simulink model "simulation"  (R2024b)
settings: Solver=ode4  StartTime=0.0  StopTime=10  FixedStep=0.001  RelTol=1e-3
settings Model: Creator=yagiz  LastModifiedBy=yagiz

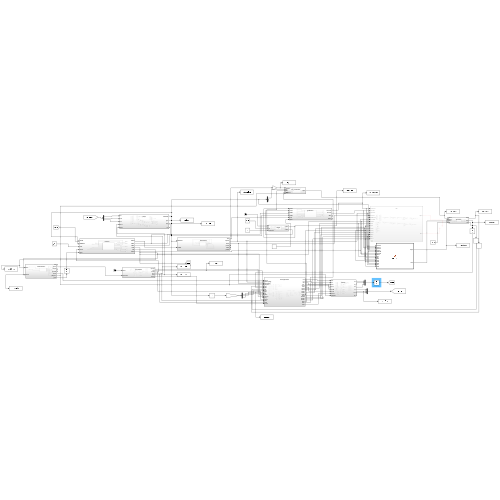
[thumbnail: Simulink's stored preview of the top-level diagram]
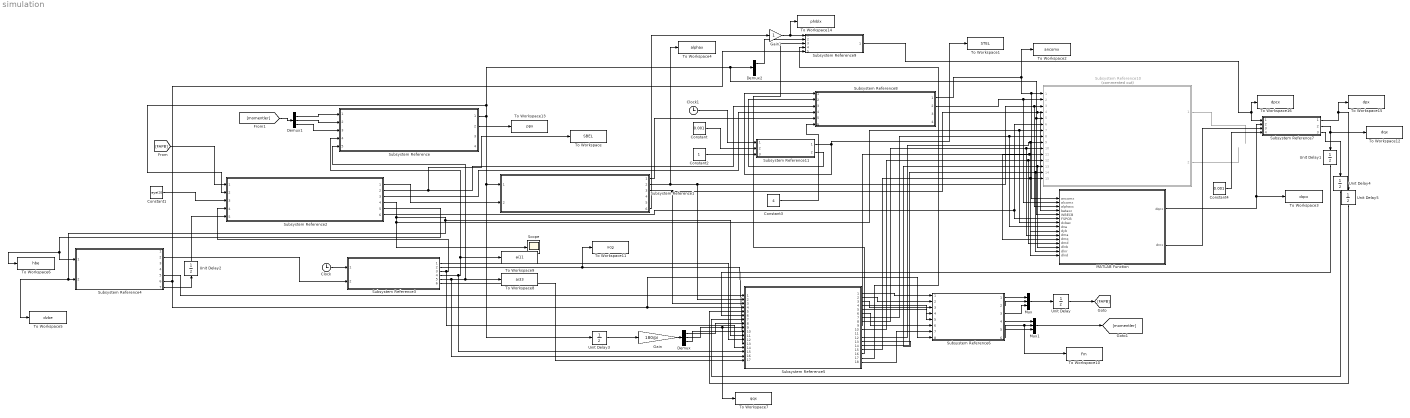
== system simulation ==
  Clock : Clock
  Clock1 : Clock
  Constant : Constant  Value=0.001
  Constant1 : Constant  Value=eye(3)
  Constant2 : Constant
  Constant3 : Constant  Value=4
  Constant4 : Constant  Value=0.001
  Demux : Demux  Outputs=3
  Demux1 : Demux  Outputs=3
  Demux2 : Demux  Outputs=3
  Gain : Gain  Gain=180/pi
  Gain1 : Gain
  MATLAB Function : MATLAB Function  TreatAsAtomicUnit=on
  Mux : Mux  Inputs=3
  Mux1 : Mux  Inputs=3
  Scope : Scope
  Subsystem Reference : Subsystem  ReferencedSubsystem=euler
  Subsystem Reference1 : Subsystem  ReferencedSubsystem=kinematics
  Subsystem Reference10 : Subsystem  Commented=on  ReferencedSubsystem=ndi
  Subsystem Reference11 : Subsystem  ReferencedSubsystem=target
  Subsystem Reference2 : Subsystem  ReferencedSubsystem=newton
  Subsystem Reference3 : Subsystem  ReferencedSubsystem=propulsion
  Subsystem Reference4 : Subsystem  ReferencedSubsystem=environment
  Subsystem Reference5 : Subsystem  ReferencedSubsystem=aerodynamics
  Subsystem Reference6 : Subsystem  ReferencedSubsystem=forces
  Subsystem Reference7 : Subsystem  ReferencedSubsystem=actuator
  Subsystem Reference8 : Subsystem  ReferencedSubsystem=guidance
  Subsystem Reference9 : Subsystem  ReferencedSubsystem=roll_controller
  To Workspace : ToWorkspace  VariableName=SBEL  SaveFormat=Timeseries  SampleTime=-1
  To Workspace1 : ToWorkspace  VariableName=STEL  SaveFormat=Timeseries  SampleTime=-1
  To Workspace10 : ToWorkspace  VariableName=Fm  SaveFormat=Timeseries  SampleTime=-1
  To Workspace11 : ToWorkspace  VariableName=xcg  SaveFormat=Timeseries  SampleTime=-1
  To Workspace12 : ToWorkspace  VariableName=dqx  SaveFormat=Timeseries  SampleTime=-1
  To Workspace13 : ToWorkspace  VariableName=ppx  SaveFormat=Timeseries  SampleTime=-1
  To Workspace14 : ToWorkspace  VariableName=phiblx  SaveFormat=Timeseries  SampleTime=-1
  To Workspace15 : ToWorkspace  VariableName=dpx  SaveFormat=Timeseries  SampleTime=-1
  To Workspace16 : ToWorkspace  VariableName=dpcx  SaveFormat=Timeseries  SampleTime=-1
  To Workspace2 : ToWorkspace  VariableName=ancomx  SaveFormat=Timeseries  SampleTime=-1
  To Workspace3 : ToWorkspace  VariableName=dqcx  SaveFormat=Timeseries  SampleTime=-1
  To Workspace4 : ToWorkspace  VariableName=alphax  SaveFormat=Timeseries  SampleTime=-1
  To Workspace5 : ToWorkspace  VariableName=dvbe  SaveFormat=Timeseries  SampleTime=-1
  To Workspace6 : ToWorkspace  VariableName=hbe  SaveFormat=Timeseries  SampleTime=-1
  To Workspace7 : ToWorkspace  VariableName=qqx  SaveFormat=Timeseries  SampleTime=-1
  To Workspace8 : ToWorkspace  VariableName=ai33  SaveFormat=Timeseries  SampleTime=-1
  To Workspace9 : ToWorkspace  VariableName=ai11  SaveFormat=Timeseries  SampleTime=-1
  Unit Delay : UnitDelay  InitialCondition=[0;0;0]  SampleTime=0.001  HasFrameUpgradeWarning=on
  Unit Delay1 : UnitDelay  SampleTime=0.001  HasFrameUpgradeWarning=on
  Unit Delay2 : UnitDelay  InitialCondition=9.8065  SampleTime=0.001  HasFrameUpgradeWarning=on
  Unit Delay3 : UnitDelay  InitialCondition=[0;0;0]  SampleTime=0.001  HasFrameUpgradeWarning=on
  Unit Delay4 : UnitDelay  SampleTime=0.001  HasFrameUpgradeWarning=on
  Unit Delay5 : UnitDelay  SampleTime=0.001  HasFrameUpgradeWarning=on
  wires:
  Constant1/1 -> Subsystem Reference2/3
  Subsystem Reference2/1 -> Subsystem Reference1/2
  Clock/1 -> Subsystem Reference3/1
  Subsystem Reference3/3 -> Subsystem Reference5/14, Subsystem Reference2/4
  Subsystem Reference3/4 -> Subsystem Reference5/15, Subsystem Reference/4, To Workspace9/1
  Subsystem Reference3/5 -> Subsystem Reference5/16, Subsystem Reference/5, To Workspace8/1
  Subsystem Reference4/2 -> Subsystem Reference3/2
  Subsystem Reference4/7 -> Unit Delay2/1
  Subsystem Reference4/5 -> Subsystem Reference5/1
  Subsystem Reference4/6 -> Subsystem Reference9/5, Subsystem Reference6/8, Subsystem Reference5/4
  Subsystem Reference1/2 -> Subsystem Reference5/2, MATLAB Function/3(alphaxc), Subsystem Reference10/3, To Workspace4/1
  Subsystem Reference1/3 -> Subsystem Reference5/3, MATLAB Function/4(betaxc), Subsystem Reference10/4
  Subsystem Reference3/6 -> Subsystem Reference5/17
  Gain/1 -> Demux/1
  Demux/1 -> Subsystem Reference5/8
  Demux/2 -> To Workspace7/1, Subsystem Reference5/9
  Demux/3 -> Subsystem Reference5/10
  Subsystem Reference3/1 -> Subsystem Reference5/12
  Subsystem Reference3/2 -> Subsystem Reference5/13, To Workspace11/1
  Subsystem Reference5/1 -> Subsystem Reference6/1
  Subsystem Reference5/2 -> Subsystem Reference6/2
  Subsystem Reference5/3 -> Subsystem Reference6/3
  Subsystem Reference5/4 -> Subsystem Reference6/4
  Subsystem Reference5/5 -> Subsystem Reference6/5
  Subsystem Reference5/6 -> Subsystem Reference6/6
  Subsystem Reference5/18 -> Subsystem Reference6/7
  Subsystem Reference6/1 -> Mux/1
  Subsystem Reference6/2 -> Mux/2
  Subsystem Reference6/3 -> Mux/3
  Mux/1 -> Unit Delay/1
  Subsystem Reference6/4 -> Mux1/1
  Subsystem Reference6/5 -> To Workspace10/1, Mux1/2
  Subsystem Reference6/6 -> Mux1/3
  [FAPB] -> Subsystem Reference2/1
  [momentler] -> Demux1/1
  Demux1/1 -> Subsystem Reference/1
  Demux1/2 -> Subsystem Reference/2
  Demux1/3 -> Subsystem Reference/3
  Subsystem Reference2/5 -> To Workspace6/1, Subsystem Reference4/1
  Unit Delay/1 -> [FAPB]
  Mux1/1 -> [momentler]
  Unit Delay2/1 -> Subsystem Reference2/5
  Subsystem Reference2/4 -> Scope/1, Subsystem Reference10/7, MATLAB Function/7(dvbec), Subsystem Reference5/11, To Workspace5/1, Subsystem Reference4/2
  Clock1/1 -> Subsystem Reference11/1
  Constant/1 -> Subsystem Reference11/2
  Constant2/1 -> Subsystem Reference11/3
  Subsystem Reference11/1 -> To Workspace1/1, Subsystem Reference8/1
  Subsystem Reference11/2 -> Subsystem Reference8/2
  Constant3/1 -> Subsystem Reference8/6
  Subsystem Reference1/1 -> Subsystem Reference8/5
  Subsystem Reference2/2 -> To Workspace/1, Subsystem Reference8/3
  Subsystem Reference2/3 -> Subsystem Reference8/4
  Subsystem Reference1/6 -> Gain1/1
  Subsystem Reference10/1 -> ?
  Subsystem Reference10/2 -> ?
  Subsystem Reference7/1 -> Unit Delay5/1, To Workspace15/1
  Subsystem Reference7/2 -> To Workspace12/1, Unit Delay1/1
  Subsystem Reference7/3 -> Unit Delay4/1
  Constant4/1 -> Subsystem Reference7/4
  Subsystem Reference8/1 -> To Workspace2/1, MATLAB Function/1(ancomx), Subsystem Reference10/1
  Subsystem Reference8/2 -> MATLAB Function/2(alcomx), Subsystem Reference10/2
  Subsystem Reference5/16 -> Subsystem Reference9/3
  Subsystem Reference5/17 -> Subsystem Reference9/4
  Subsystem Reference5/7 -> Subsystem Reference10/8, MATLAB Function/8(dna)
  Subsystem Reference5/12 -> MATLAB Function/9(dyb), Subsystem Reference10/9
  Subsystem Reference5/8 -> MATLAB Function/10(dma), Subsystem Reference10/10
  Subsystem Reference5/9 -> MATLAB Function/11(dmq), Subsystem Reference10/11
  Subsystem Reference5/10 -> MATLAB Function/12(dmd), Subsystem Reference10/12
  Subsystem Reference5/13 -> MATLAB Function/13(dlnb), Subsystem Reference10/13
  Subsystem Reference5/14 -> MATLAB Function/14(dlnr), Subsystem Reference10/14
  Subsystem Reference5/15 -> MATLAB Function/15(dlnd), Subsystem Reference10/15
  Subsystem Reference/1 -> MATLAB Function/5(WBECB), Subsystem Reference10/5, Demux2/1, Subsystem Reference2/2, Unit Delay3/1, Subsystem Reference1/1
  Subsystem Reference2/6 -> Subsystem Reference10/6, MATLAB Function/6(FSPCB)
  MATLAB Function/1(dqcx) -> Subsystem Reference7/2, To Workspace3/1
  MATLAB Function/2(drcx) -> Subsystem Reference7/3
  Unit Delay3/1 -> Gain/1
  Subsystem Reference/2 -> To Workspace13/1
  Subsystem Reference9/1 -> To Workspace16/1, Subsystem Reference7/1
  Demux2/1 -> Subsystem Reference9/2
  Gain1/1 -> To Workspace14/1, Subsystem Reference9/1
  Unit Delay1/1 -> Subsystem Reference5/6
  Unit Delay4/1 -> Subsystem Reference5/7
  Unit Delay5/1 -> Subsystem Reference5/5

== matlab function simulation/MATLAB Function ==
  data: ancomx input; dqcx output; alcomx input; alphaxc input; betaxc input; WBECB input; FSPCB input; dvbec input; dna input; dyb input; dma input; dmq input; dmd input; dlnb input; dlnr input; dlnd input; drcx output
function [dqcx, drcx] = ndi_fcn(ancomx, alcomx, alphaxc, betaxc, ...
    WBECB, FSPCB, dvbec, dna, dyb, dma, dmq, dmd, dlnb, dlnr, dlnd)

% NDI autopilot — matches control_ndi() in control.py exactly

dqcx = 0.0;
drcx = 0.0;

AGRAV  = 9.80665;
RAD    = pi / 180.0;
DEG    = 180.0 / pi;
SMALL  = 1e-7;

% Config constants (from workspace)
wn_ndi_q = 50.0;
wn_ndi_r = 50.0;
k_alpha  = 10.0;
k_beta   = 10.0;
dqlimx   = 28.0;
drlimx   = 28.0;
wblimx   = 30.0 * RAD;
alplimx  = 46.0 * RAD;
alimit   = 50.0;

q = WBECB(2);
r = WBECB(3);

fspb2 =  FSPCB(2);
fspb3 =  FSPCB(3);

an_meas = -fspb3 / AGRAV;
al_meas =  fspb2 / AGRAV;

alpha = alphaxc * RAD;
beta  = betaxc  * RAD;

% Structural accel limit
aa = sqrt(ancomx^2 + alcomx^2);
if aa > alimit
    if abs(ancomx) < SMALL && abs(alcomx) < SMALL
        phi = 0.0;
    else
        phi = atan2(ancomx, alcomx);
    end
    alcomx = aa * cos(phi);
    ancomx = aa * sin(phi);
end

% STEP 1: Force inversion
if abs(dna) > SMALL
    dna_s = dna;
else
    if dna >= 0; dna_s = SMALL; else; dna_s = -SMALL; end
end
if abs(dyb) > SMALL
    dyb_s = dyb;
else
    if dyb >= 0; dyb_s = SMALL; else; dyb_s = -SMALL; end
end

alpha_cmd = AGRAV * ancomx / dna_s;
beta_cmd  = AGRAV * alcomx / dyb_s;
alpha_cmd = max(min(alpha_cmd,  alplimx), -alplimx);
beta_cmd  = max(min(beta_cmd,   alplimx), -alplimx);

% STEP 2: Kinematic inversion
V_safe = max(dvbec, 30.0);
q_cmd = k_alpha * (alpha_cmd - alpha) + AGRAV * an_meas / V_safe;
r_cmd = k_beta  * (beta - beta_cmd)   + AGRAV * al_meas / V_safe;
q_cmd = max(min(q_cmd,  wblimx), -wblimx);
r_cmd = max(min(r_cmd,  wblimx), -wblimx);

% STEP 3: Inner NDI
q_dot_des = wn_ndi_q * (q_cmd - q);
r_dot_des = wn_ndi_r * (r_cmd - r);

q_dot_model = dma * alpha + dmq * q;
r_dot_model = dlnb * beta + dlnr * r;

if abs(dmd) > SMALL
    dmd_s = dmd;
else
    if dmd >= 0; dmd_s = -SMALL; else; dmd_s = -SMALL; end
end
if abs(dlnd) > SMALL
    dlnd_s = dlnd;
else
    if dlnd >= 0; dlnd_s = -SMALL; else; dlnd_s = -SMALL; end
end

dqc = (q_dot_des - q_dot_model) / dmd_s;
drc = (r_dot_des - r_dot_model) / dlnd_s;

dqcx = max(min(dqc * DEG,  dqlimx), -dqlimx);
drcx = max(min(drc * DEG,  drlimx), -drlimx);
